simulink model "two_area_model"  (R2020a)
settings: Solver=VariableStepAuto  StartTime=0.0  StopTime=10.0  RelTol=1e-3
values from neighbouring files (symbols this model uses):
  ExpandSmachs = zeros(Nbus,NSmachs)    [Synch_parameter_gen_base.m]    (also in Synch_parameter_sys_base.m)
  machine_base_mva = mac_con(:,2)    [Synch_parameter_gen_base.m]    (also in Synch_parameter_sys_base.m)
  s_D = mac_con(:,16)    [Synch_parameter_gen_base.m]    (also in Synch_parameter_sys_base.m = mac_con(:,16).*system_base_mva./machine_base_mva)
  s_delta = angle(s_Eq)    [generic_Sync_Init.m]
  s_Edd = -(s_xq - s_xqd).*s_iq    [generic_Sync_Init.m]
  s_Efd = abs(s_Eq)-(s_xd-s_xq).*s_id    [generic_Sync_Init.m]
  s_Eqd = s_Efd+ (s_xd - s_xdd).*s_id    [generic_Sync_Init.m]
  s_H = mac_con(:,15)    [Synch_parameter_gen_base.m]    (also in Synch_parameter_sys_base.m = mac_con(:,15).*system_base_mva./machine_base_mva)
  s_Ka = 200    [four_mac_data.m]    (also in two_area_synch.m)
  s_Psi1d = s_Eqd+(s_xdd - s_xls).*s_id    [generic_Sync_Init.m]
  s_Psi2q = -s_Edd+(s_xqd - s_xls).*s_iq    [generic_Sync_Init.m]
  s_Rgov = s_Rgov    [Synch_parameter_gen_base.m]    (also in Synch_parameter_sys_base.m = s_Rgov.*system_base_mva./machine_base_mva; four_mac_data.m = 0.05; two_area_synch.m = 0.05)
  s_Rs = mac_con(:,4)    [Synch_parameter_gen_base.m]    (also in Synch_parameter_sys_base.m = mac_con(:,4).*system_base_mva./machine_base_mva)
  s_Ta = 0.02    [four_mac_data.m]    (also in two_area_synch.m)
  s_Tdod = mac_con(:,8)    [Synch_parameter_gen_base.m]    (also in Synch_parameter_sys_base.m)
  s_Tdodd = mac_con(:,9)    [Synch_parameter_gen_base.m]    (also in Synch_parameter_sys_base.m)
  s_Tg = 0.2    [four_mac_data.m]    (also in two_area_synch.m)
  s_Tm = s_Te    [generic_Sync_Init.m]
  s_Tqod = mac_con(:,13)    [Synch_parameter_gen_base.m]    (also in Synch_parameter_sys_base.m)
  s_Tqodd = mac_con(:,14)    [Synch_parameter_gen_base.m]    (also in Synch_parameter_sys_base.m)
  s_Vref = s_volt+1./s_Ka.*s_Efd    [generic_Sync_Init.m]
  s_wb = 2*pi*s_f    (= 376.991118431)    [generic_Sync_Init.m]
  s_ws = 1    [generic_Sync_Init.m]
  s_xd = mac_con(:,5)    [Synch_parameter_gen_base.m]    (also in Synch_parameter_sys_base.m = mac_con(:,5).*system_base_mva./machine_base_mva)
  s_xdd = mac_con(:,6)    [Synch_parameter_gen_base.m]    (also in Synch_parameter_sys_base.m = mac_con(:,6).*system_base_mva./machine_base_mva)
  s_xddd = mac_con(:,7)    [Synch_parameter_gen_base.m]    (also in Synch_parameter_sys_base.m = mac_con(:,7).*system_base_mva./machine_base_mva)
  s_xls = mac_con(:,3)    [Synch_parameter_gen_base.m]    (also in Synch_parameter_sys_base.m = mac_con(:,3).*system_base_mva./machine_base_mva)
  s_xq = mac_con(:,10)    [Synch_parameter_gen_base.m]    (also in Synch_parameter_sys_base.m = mac_con(:,10).*system_base_mva./machine_base_mva)
  s_xqd = mac_con(:,11)    [Synch_parameter_gen_base.m]    (also in Synch_parameter_sys_base.m = mac_con(:,11).*system_base_mva./machine_base_mva)
  s_xqdd = mac_con(:,12)    [Synch_parameter_gen_base.m]    (also in Synch_parameter_sys_base.m = mac_con(:,12).*system_base_mva./machine_base_mva)
  SelectSmachs = zeros(NSmachs,Nbus)    [Synch_parameter_gen_base.m]    (also in Synch_parameter_sys_base.m)
  system_base_mva = 100    [four_mac_data.m]    (also in four_mac_run.m; two_area_synch.m)
  Z = inv(Y)    [four_mac_data.m]    (also in four_mac_run.m; two_area_synch.m)
undefined symbols (not defined in the file or in its folder): j
settings Model: Creator=lenovo  LastModifiedBy=EBUKA
settings OptimizationCC: LifeSpan=inf
settings DebuggingCC: ArithmeticOperatorsInVariantConditions=warning
settings SFSimCC: CustomCodeUndefinedFunction=UseInterfaceOnly
settings CodeAppCC: StateflowObjectComments=on
settings SimscapeCC: SimscapeNormalizeSystem=off

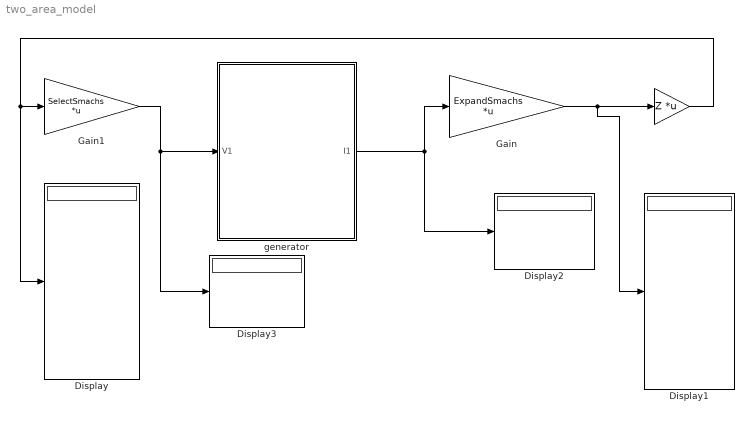
== system two_area_model ==
  "       " : Gain  Gain=Z  Multiplication=Matrix(K*u)
  Display{,1..3} (4 alike) : Display
  Gain : Gain  Gain=ExpandSmachs  Multiplication=Matrix(K*u)
  Gain1 : Gain  Gain=SelectSmachs  Multiplication=Matrix(K*u)
  generator : Subsystem
  wires:
  generator/1(I1) -> Gain/1, Display2/1
  Gain/1 -> Display1/1, "       "/1
  Gain1/1 -> Display3/1, generator/1(V1)
  "       "/1 -> Display/1, Gain1/1

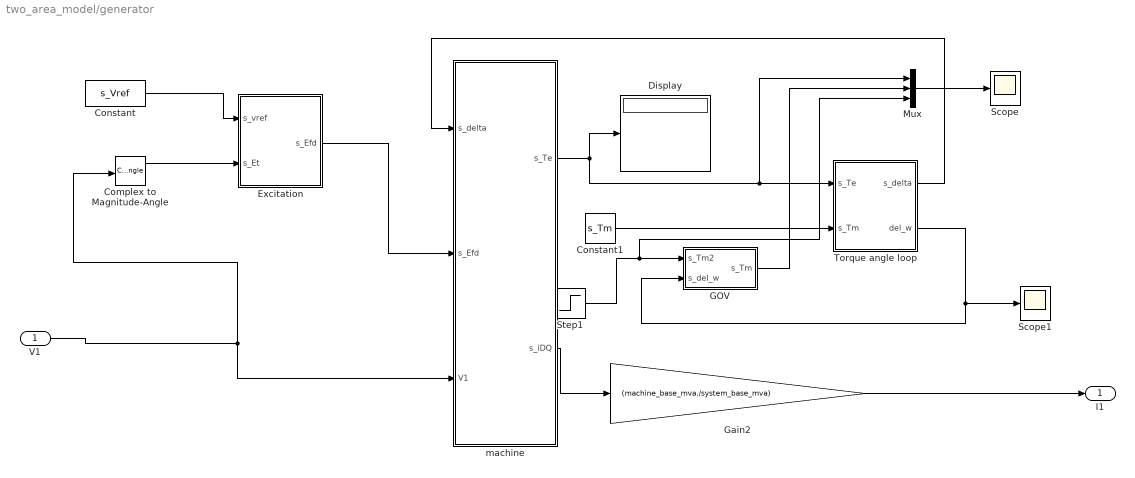
== system two_area_model/generator ==
  V1 : Inport
  Complex to Magnitude-Angle : ComplexToMagnitudeAngle
  Constant : Constant  Value=s_Vref
  Constant1 : Constant  Value=s_Tm
  Display : Display
  Excitation : Subsystem
  GOV : Subsystem
  Gain2 : Gain  Gain=(machine_base_mva./system_base_mva)
  Mux : Mux  Inputs=3
  Scope : Scope
  Scope1 : Scope
  Step1 : Step  Before=0.7792  After=s_Tm  SampleTime=0
  Torque angle loop : Subsystem
  machine : Subsystem
  I1 : Outport
  wires:
  machine/1(s_Te) -> Display/1, Mux/1, Torque angle loop/1(s_Te)
  V1/1 -> machine/3(V1), Complex to Magnitude-Angle/1
  Complex to Magnitude-Angle/1 -> Excitation/2(s_Et)
  Gain2/1 -> I1/1
  Excitation/1(s_Efd) -> machine/2(s_Efd)
  Torque angle loop/2(del_w) -> Scope1/1, GOV/2(s_del_w)
  Constant/1 -> Excitation/1(s_vref)
  Torque angle loop/1("s_delta ") -> machine/1("s_delta ")
  Mux/1 -> Scope/1
  machine/2(s_iDQ) -> Gain2/1
  Step1/1 -> Mux/3, GOV/1(s_Tm2)
  Constant1/1 -> Torque angle loop/2(s_Tm)
  GOV/1(s_Tm) -> Mux/2

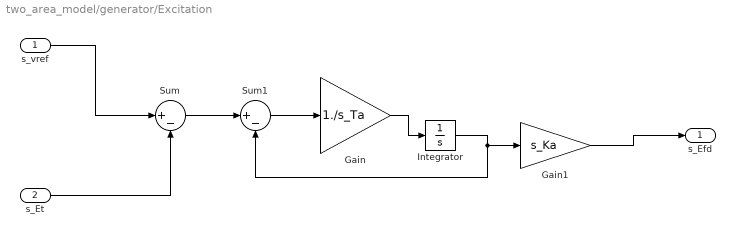
== system two_area_model/generator/Excitation ==
  s_vref : Inport
  s_Et : Inport  Port=2
  Gain : Gain  Gain=1./s_Ta
  Gain1 : Gain  Gain=s_Ka
  Integrator : Integrator  InitialCondition=s_Efd./s_Ka
  Sum : Sum  Inputs=|+-
  Sum1 : Sum  Inputs=|+-
  s_Efd : Outport
  wires:
  s_vref/1 -> Sum/1
  s_Et/1 -> Sum/2
  Sum/1 -> Sum1/1
  Sum1/1 -> Gain/1
  Gain/1 -> Integrator/1
  Integrator/1 -> Sum1/2, Gain1/1
  Gain1/1 -> s_Efd/1

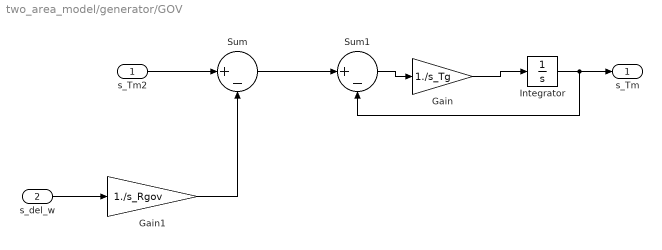
== system two_area_model/generator/GOV ==
  s_Tm2 : Inport
  s_del_w : Inport  Port=2
  Gain : Gain  Gain=1./s_Tg
  Gain1 : Gain  Gain=1./s_Rgov
  Integrator : Integrator  InitialCondition=s_Tm
  Sum : Sum  Inputs=|+-
  Sum1 : Sum  Inputs=|+-
  s_Tm : Outport
  wires:
  s_Tm2/1 -> Sum/1
  s_del_w/1 -> Gain1/1
  Sum/1 -> Sum1/1
  Sum1/1 -> Gain/1
  Gain/1 -> Integrator/1
  Integrator/1 -> Sum1/2, s_Tm/1
  Gain1/1 -> Sum/2

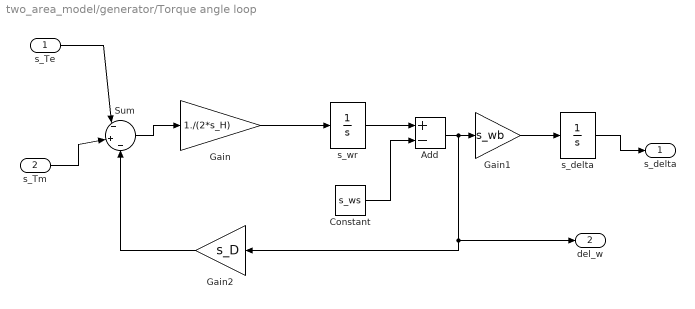
== system two_area_model/generator/Torque angle loop ==
  s_Te : Inport
  s_Tm : Inport  Port=2
  Add : Sum  Inputs=+-
  Constant : Constant  Value=s_ws
  Gain : Gain  Gain=1./(2*s_H)
  Gain1 : Gain  Gain=s_wb
  Gain2 : Gain  Gain=s_D
  Sum : Sum  Inputs=|-|+|-
  s_delta : Integrator  InitialCondition=s_delta
  s_wr : Integrator  InitialCondition=s_ws
  "s_delta " : Outport
  del_w : Outport  Port=2
  wires:
  s_Tm/1 -> Sum/2
  Gain/1 -> s_wr/1
  s_delta/1 -> "s_delta "/1
  Constant/1 -> Add/2
  Sum/1 -> Gain/1
  s_wr/1 -> Add/1
  Gain1/1 -> s_delta/1
  Gain2/1 -> Sum/3
  Add/1 -> del_w/1, Gain2/1, Gain1/1
  s_Te/1 -> Sum/1

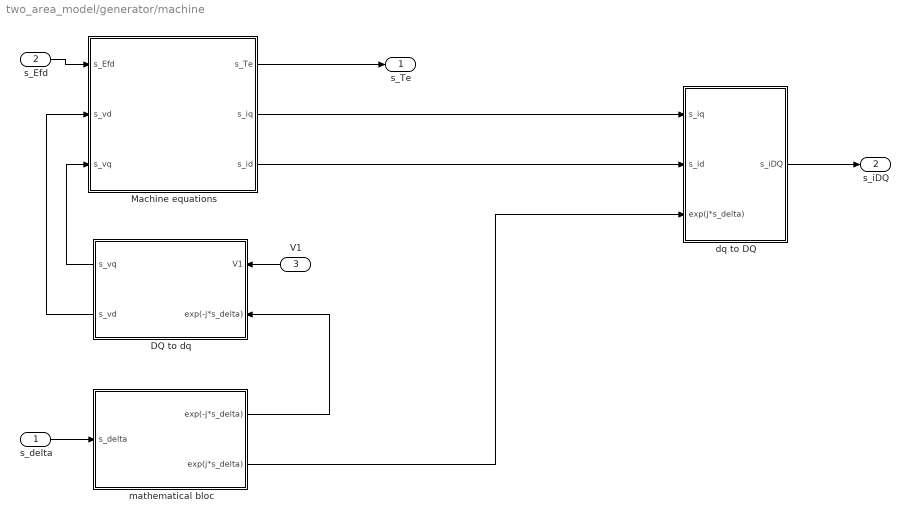
== system two_area_model/generator/machine ==
  "s_delta " : Inport
  s_Efd : Inport  Port=2
  V1 : Inport  Port=3
  DQ to dq : Subsystem
  Machine equations : Subsystem
  dq to DQ : Subsystem
  mathematical bloc : Subsystem
  s_Te : Outport
  s_iDQ : Outport  Port=2
  wires:
  "s_delta "/1 -> mathematical bloc/1("s_delta ")
  Machine equations/1(s_Te) -> s_Te/1
  s_Efd/1 -> Machine equations/1(s_Efd)
  V1/1 -> DQ to dq/1(V1)
  DQ to dq/1(s_vq) -> Machine equations/3(s_vq)
  DQ to dq/2(s_vd) -> Machine equations/2(s_vd)
  mathematical bloc/1(exp(-j*s_delta)) -> DQ to dq/2("exp(-j*s_delta) ")
  mathematical bloc/2(exp(j*s_delta)) -> dq to DQ/3(exp(j*s_delta))
  Machine equations/2(s_iq) -> dq to DQ/1(s_iq)
  Machine equations/3(s_id) -> dq to DQ/2(s_id)
  dq to DQ/1(s_iDQ) -> s_iDQ/1

== system two_area_model/generator/machine/DQ to dq ==
  V1 : Inport
  "exp(-j*s_delta) " : Inport  Port=2
  Complex to Real-Imag : ComplexToRealImag
  Product : Product
  s_vq : Outport
  s_vd : Outport  Port=2
  wires:
  "exp(-j*s_delta) "/1 -> Product/2
  V1/1 -> Product/1
  Product/1 -> Complex to Real-Imag/1
  Complex to Real-Imag/1 -> s_vq/1
  Complex to Real-Imag/2 -> s_vd/1

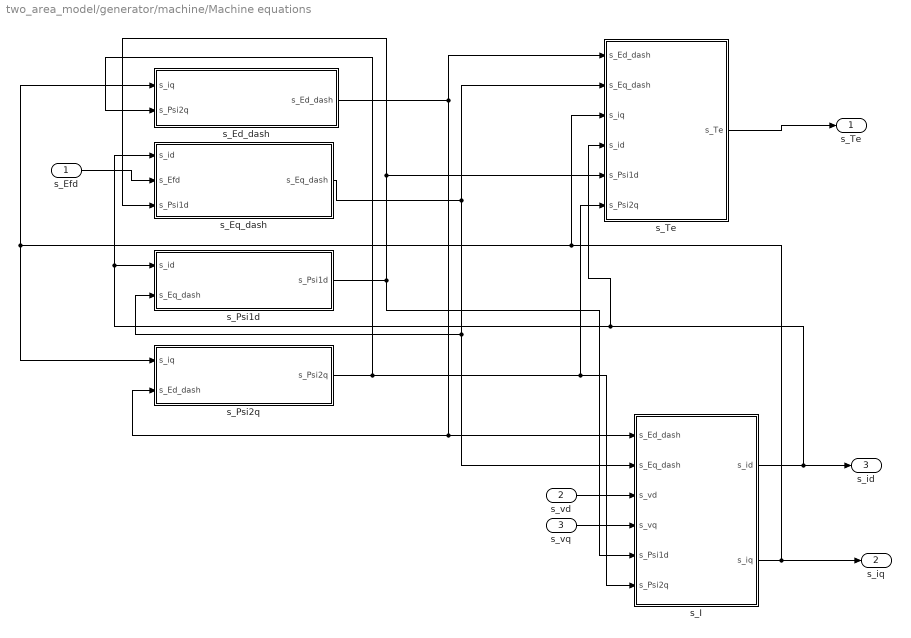
== system two_area_model/generator/machine/Machine equations ==
  s_Efd : Inport
  s_vd : Inport  Port=2
  s_vq : Inport  Port=3
  s_Ed_dash : Subsystem
  s_Eq_dash : Subsystem
  s_I : Subsystem
  s_Psi1d : Subsystem
  s_Psi2q : Subsystem
  "s_Te " : Subsystem
  s_Te : Outport
  s_iq : Outport  Port=2
  s_id : Outport  Port=3
  wires:
  s_Efd/1 -> s_Eq_dash/2(s_Efd)
  s_vd/1 -> s_I/3(s_vd)
  s_vq/1 -> s_I/4(s_vq)
  s_I/1(s_id) -> "s_Te "/4(s_id), s_Eq_dash/1(s_id), s_Psi1d/1(s_id), s_id/1
  s_I/2(s_iq) -> s_iq/1, "s_Te "/3(s_iq), s_Psi2q/1(s_iq), s_Ed_dash/1(s_iq)
  "s_Te "/1(s_Te) -> s_Te/1
  s_Ed_dash/1("s_Ed_dash ") -> "s_Te "/1("s_Ed_dash "), s_Psi2q/2("s_Ed_dash    "), s_I/1("s_Ed_dash  ")
  s_Eq_dash/1(s_Eq_dash) -> "s_Te "/2("s_Eq_dash "), s_I/2(s_Eq_dash), s_Psi1d/2(s_Eq_dash)
  s_Psi1d/1(s_Psi1d) -> s_I/5(s_Psi1d), "s_Te "/5(s_Psi1d), s_Eq_dash/3(s_Psi1d)
  s_Psi2q/1(s_Psi2q) -> "s_Te "/6(s_Psi2q), s_I/6(s_Psi2q), s_Ed_dash/2(s_Psi2q)

== system two_area_model/generator/machine/dq to DQ ==
  s_iq : Inport
  s_id : Inport  Port=2
  exp(j*s_delta) : Inport  Port=3
  Product : Product
  Real-Imag to Complex : RealImagToComplex
  s_iDQ : Outport
  wires:
  s_iq/1 -> Real-Imag to Complex/1
  s_id/1 -> Real-Imag to Complex/2
  Real-Imag to Complex/1 -> Product/1
  exp(j*s_delta)/1 -> Product/2
  Product/1 -> s_iDQ/1

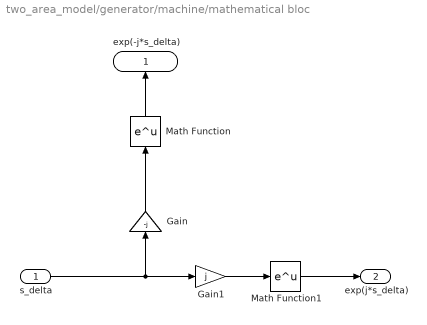
== system two_area_model/generator/machine/mathematical bloc ==
  "s_delta " : Inport
  Gain : Gain  Gain=-j
  Gain1 : Gain  Gain=j
  Math Function : Math  SignedPower=on  SaturateOnIntegerOverflow=on
  Math Function1 : Math  SignedPower=on  SaturateOnIntegerOverflow=on
  exp(-j*s_delta) : Outport
  exp(j*s_delta) : Outport  Port=2
  wires:
  Gain/1 -> Math Function/1
  Math Function/1 -> exp(-j*s_delta)/1
  "s_delta "/1 -> Gain1/1, Gain/1
  Gain1/1 -> Math Function1/1
  Math Function1/1 -> exp(j*s_delta)/1

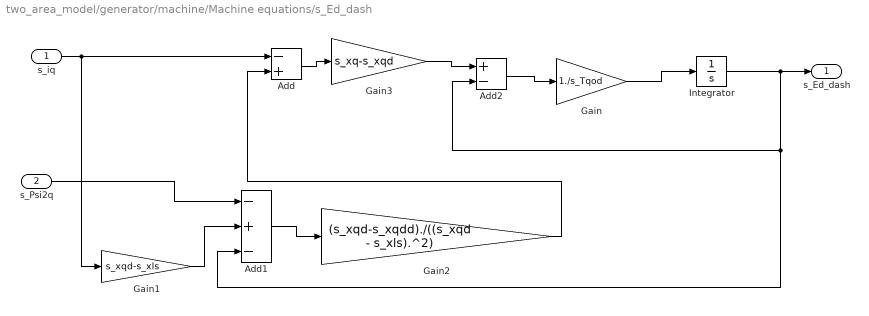
== system two_area_model/generator/machine/Machine equations/s_Ed_dash ==
  s_iq : Inport
  s_Psi2q : Inport  Port=2
  Add : Sum  Inputs=-+
  Add1 : Sum  Inputs=-+-
  Add2 : Sum  Inputs=+-
  Gain : Gain  Gain=1./s_Tqod
  Gain1 : Gain  Gain=s_xqd-s_xls
  Gain2 : Gain  Gain=(s_xqd-s_xqdd)./((s_xqd - s_xls).^2)
  Gain3 : Gain  Gain=s_xq-s_xqd
  Integrator : Integrator  InitialCondition=s_Edd
  "s_Ed_dash " : Outport
  wires:
  Add1/1 -> Gain2/1
  Gain/1 -> Integrator/1
  Gain1/1 -> Add1/2
  Gain2/1 -> Add/2
  Integrator/1 -> Add1/3, Add2/2, "s_Ed_dash "/1
  Add/1 -> Gain3/1
  s_iq/1 -> Add/1, Gain1/1
  s_Psi2q/1 -> Add1/1
  Gain3/1 -> Add2/1
  Add2/1 -> Gain/1

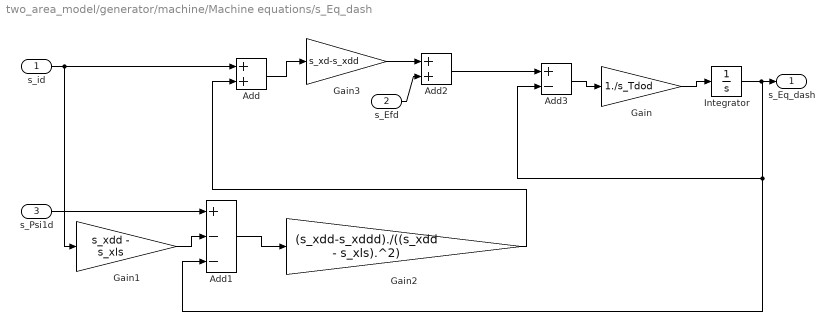
== system two_area_model/generator/machine/Machine equations/s_Eq_dash ==
  s_id : Inport
  s_Efd : Inport  Port=2
  s_Psi1d : Inport  Port=3
  Add : Sum
  Add1 : Sum  Inputs=+--
  Add2 : Sum
  Add3 : Sum  Inputs=+-
  Gain : Gain  Gain=1./s_Tdod
  Gain1 : Gain  Gain=s_xdd - s_xls
  Gain2 : Gain  Gain=(s_xdd-s_xddd)./((s_xdd - s_xls).^2)
  Gain3 : Gain  Gain=s_xd-s_xdd
  Integrator : Integrator  InitialCondition=s_Eqd
  s_Eq_dash : Outport
  wires:
  Add1/1 -> Gain2/1
  Gain/1 -> Integrator/1
  Gain1/1 -> Add1/2
  Gain2/1 -> Add/2
  Integrator/1 -> s_Eq_dash/1, Add1/3, Add3/2
  Add/1 -> Gain3/1
  s_id/1 -> Add/1, Gain1/1
  s_Psi1d/1 -> Add1/1
  s_Efd/1 -> Add2/2
  Gain3/1 -> Add2/1
  Add2/1 -> Add3/1
  Add3/1 -> Gain/1

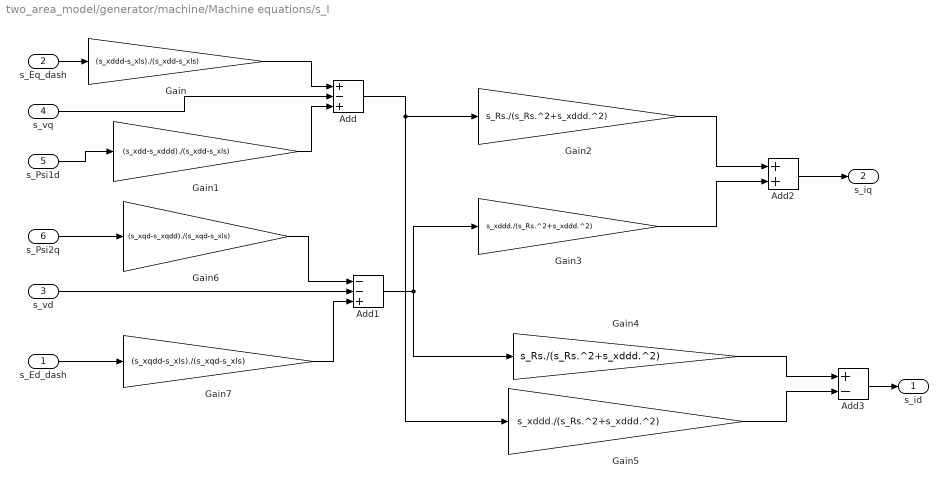
== system two_area_model/generator/machine/Machine equations/s_I ==
  "s_Ed_dash  " : Inport
  s_Eq_dash : Inport  Port=2
  s_vd : Inport  Port=3
  s_vq : Inport  Port=4
  s_Psi1d : Inport  Port=5
  s_Psi2q : Inport  Port=6
  Add : Sum  Inputs=+-+
  Add1 : Sum  Inputs=--+
  Add2 : Sum
  Add3 : Sum  Inputs=+-
  Gain : Gain  Gain=(s_xddd-s_xls)./(s_xdd-s_xls)
  Gain1 : Gain  Gain=(s_xdd-s_xddd)./(s_xdd-s_xls)
  Gain2 : Gain  Gain=s_Rs./(s_Rs.^2+s_xddd.^2)
  Gain3 : Gain  Gain=s_xddd./(s_Rs.^2+s_xddd.^2)
  Gain4 : Gain  Gain=s_Rs./(s_Rs.^2+s_xddd.^2)
  Gain5 : Gain  Gain=s_xddd./(s_Rs.^2+s_xddd.^2)
  Gain6 : Gain  Gain=(s_xqd-s_xqdd)./(s_xqd-s_xls)
  Gain7 : Gain  Gain=(s_xqdd-s_xls)./(s_xqd-s_xls)
  s_id : Outport
  s_iq : Outport  Port=2
  wires:
  s_Eq_dash/1 -> Gain/1
  Gain/1 -> Add/1
  s_vq/1 -> Add/2
  s_Psi1d/1 -> Gain1/1
  Gain1/1 -> Add/3
  Add/1 -> Gain5/1, Gain2/1
  Gain2/1 -> Add2/1
  Add2/1 -> s_iq/1
  Add1/1 -> Gain3/1, Gain4/1
  Gain3/1 -> Add2/2
  Add3/1 -> s_id/1
  Gain4/1 -> Add3/1
  Gain5/1 -> Add3/2
  s_Psi2q/1 -> Gain6/1
  Gain6/1 -> Add1/1
  s_vd/1 -> Add1/2
  Gain7/1 -> Add1/3
  "s_Ed_dash  "/1 -> Gain7/1

== system two_area_model/generator/machine/Machine equations/s_Psi1d ==
  s_id : Inport
  s_Eq_dash : Inport  Port=2
  Add : Sum  Inputs=++-
  Gain : Gain  Gain=s_xdd-s_xls
  Gain1 : Gain  Gain=1./s_Tdodd
  Integrator : Integrator  InitialCondition=s_Psi1d
  s_Psi1d : Outport
  wires:
  Integrator/1 -> Add/3, s_Psi1d/1
  Gain1/1 -> Integrator/1
  Add/1 -> Gain1/1
  s_id/1 -> Gain/1
  Gain/1 -> Add/1
  s_Eq_dash/1 -> Add/2

== system two_area_model/generator/machine/Machine equations/s_Psi2q ==
  s_iq : Inport
  "s_Ed_dash    " : Inport  Port=2
  Add : Sum  Inputs=+--
  Gain : Gain  Gain=s_xqd-s_xls
  Gain1 : Gain  Gain=1./s_Tqodd
  Integrator : Integrator  InitialCondition=s_Psi2q
  s_Psi2q : Outport
  wires:
  Gain/1 -> Add/1
  "s_Ed_dash    "/1 -> Add/2
  Gain1/1 -> Integrator/1
  s_iq/1 -> Gain/1
  Add/1 -> Gain1/1
  Integrator/1 -> s_Psi2q/1, Add/3

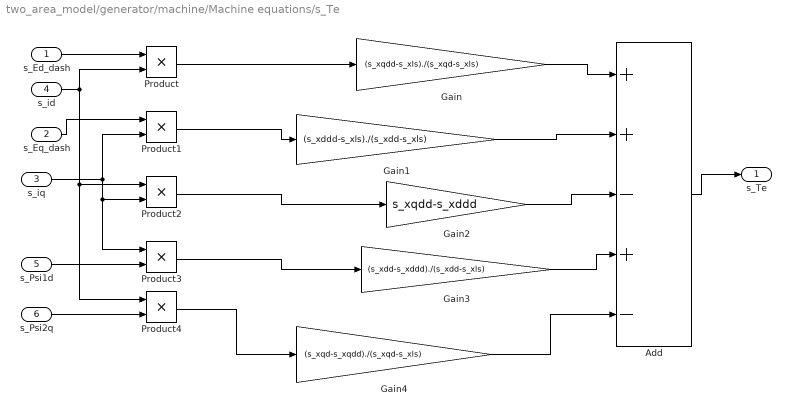
== system two_area_model/generator/machine/Machine equations/s_Te  ==
  "s_Ed_dash " : Inport
  "s_Eq_dash " : Inport  Port=2
  s_iq : Inport  Port=3
  s_id : Inport  Port=4
  s_Psi1d : Inport  Port=5
  s_Psi2q : Inport  Port=6
  Add : Sum  Inputs=++-+-
  Gain : Gain  Gain=(s_xqdd-s_xls)./(s_xqd-s_xls)
  Gain1 : Gain  Gain=(s_xddd-s_xls)./(s_xdd-s_xls)
  Gain2 : Gain  Gain=s_xqdd-s_xddd
  Gain3 : Gain  Gain=(s_xdd-s_xddd)./(s_xdd-s_xls)
  Gain4 : Gain  Gain=(s_xqd-s_xqdd)./(s_xqd-s_xls)
  Product{,1..4} (5 alike) : Product
  s_Te : Outport
  wires:
  "s_Ed_dash "/1 -> Product/1
  s_id/1 -> Product4/1, Product2/1, Product/2
  "s_Eq_dash "/1 -> Product1/1
  s_iq/1 -> Product1/2, Product2/2, Product3/1
  s_Psi1d/1 -> Product3/2
  s_Psi2q/1 -> Product4/2
  Product/1 -> Gain/1
  Product1/1 -> Gain1/1
  Product2/1 -> Gain2/1
  Product3/1 -> Gain3/1
  Product4/1 -> Gain4/1
  Add/1 -> s_Te/1
  Gain/1 -> Add/1
  Gain1/1 -> Add/2
  Gain2/1 -> Add/3
  Gain3/1 -> Add/4
  Gain4/1 -> Add/5
